simulink model "engine_model"  (R2022b)
settings: Solver=ode3  StartTime=0.0  StopTime=10  FixedStep=0.0005  RelTol=1e-3  EnableMultiTasking=on
undefined symbols (not defined in the file): sigbuilder_block
settings Model: Creator=Administrator  LastModifiedBy=Mr.Eastern
settings SolverCC: AllowMultiTaskInputOutput=on  AlgebraicLoopSolver=TrustRegion
settings DataIOCC: LimitDataPoints=on  SaveFormat=Array  SignalLoggingSaveFormat=ModelDataLogs  ReturnWorkspaceOutputs=off
settings OptimizationCC: ExpressionDepthLimit=2147483647  InitFltsAndDblsToZero=on  LifeSpan=inf
settings DebuggingCC: SaveWithParameterizedLinksMsg=none  UnderspecifiedInitializationDetection=Classic  MergeDetectMultiDrivingBlocksExec=none  SolverPrmCheckMsg=warning  FcnCallInpInsideContextMsg=warning  UnconnectedInputMsg=warning  UnconnectedOutputMsg=warning  UnconnectedLineMsg=warning  StateNameClashWarn=warning  SFUnexpectedBacktrackingDiag=warning  SFNoUnconditionalDefaultTransitionDiag=warning  SFExecutionAtInitializationDiag=none  SFMachineParentedDataDiag=warning  ArithmeticOperatorsInVariantConditions=warning
settings HardwareCC: ProdBitPerPointer=32  ProdBitPerSizeT=32  ProdBitPerPtrDiffT=32  ProdLargestAtomicFloat=None  ProdIntDivRoundTo=Undefined  ProdEndianess=Unspecified  ProdWordSize=32  ProdHWDeviceType=32-bit Generic
settings ModelReferenceCC: PropagateSignalLabelsOutOfModel=off
settings CodeAppCC: StateflowObjectComments=on
settings GRTTargetCC: TargetFcnLib=ansi_tfl_tmw.mat  TargetLangStandard=C89/C90 (ANSI)  CombineOutputUpdateFcns=off  GRTInterface=on
settings ConfigComp: CovMetricSettings=dw  CovSaveCumulativeToWorkspaceVar=on  CovSaveSingleToWorkspaceVar=on

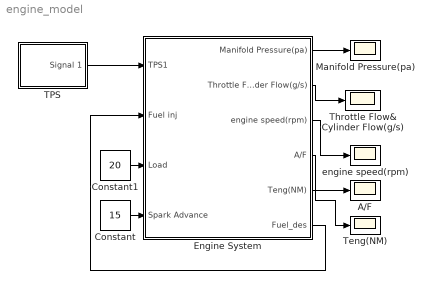
== system engine_model ==
  A/F : Scope
  Constant : Constant  Value=15
  Constant1 : Constant  Value=20
  Engine System : Subsystem
  Manifold Pressure(pa) : Scope
  TPS : Subsystem  Tag=STV Subsys  LoadFcn=sigbuilder_block('load');  StartFcn=sigbuilder_block('start');  StopFcn=sigbuilder_block('stop');  ClipboardFcn=sigbuilder_block('clipboard');  mask(Sigbuilder block){tuvar=[0:10]}
      mask help: Sigbuilder GUI
      mask init:
      | if ~strcmp(get_param(bdroot(gcb),'SimulationStatus'),'stopped') tuvar = sigbuilder_block('maskInit'); end
      settings: CopyFcn=sigbuilder_block('copy');  DeleteFcn=sigbuilder_block('delete');  ModelCloseFcn=sigbuilder_block('modelClose');  PreSaveFcn=sigbuilder_block('preSave');  PauseFcn=sigbuilder_block('pause')  ContinueFcn=sigbuilder_block('continue')  NameChangeFcn=sigbuilder_block('namechange');  OpenFcn=sigbuilder_block('open',[1520 218.5 535 348.5 ]);  CloseFcn=sigbuilder_block('close');
      mask Display: plot(0, 0, 100, 100,[2, 2, 32, 32, 2], [68, 8, 8, 68, 68],[32, 2], [38, 38], [32, 19, 2],[53, 60, 44], [32, 17, 17, 2],[16, 16, 31, 31]);txt = getActiveGroup(gcbh);text(2, 100, txt,'verticalAlignment', 'top');
  Teng(NM) : Scope
  Throttle Flow& Cylinder Flow(g/s) : Scope
  engine speed(rpm) : Scope
  wires:
  Constant/1 -> Engine System/4(Spark Advance)
  Engine System/6(Fuel_des) -> Engine System/2(Fuel inj)
  Engine System/1(Manifold Pressure(pa)) -> Manifold Pressure(pa)/1
  Engine System/2(Throttle Flow& Cylinder Flow(g/s)) -> Throttle Flow& Cylinder Flow(g/s)/1
  Engine System/3(engine speed(rpm)) -> engine speed(rpm)/1
  Engine System/4(A/F) -> A/F/1
  Engine System/5(Teng(NM)) -> Teng(NM)/1
  Constant1/1 -> Engine System/3(Load)
  TPS/1(Signal 1) -> Engine System/1(TPS1)

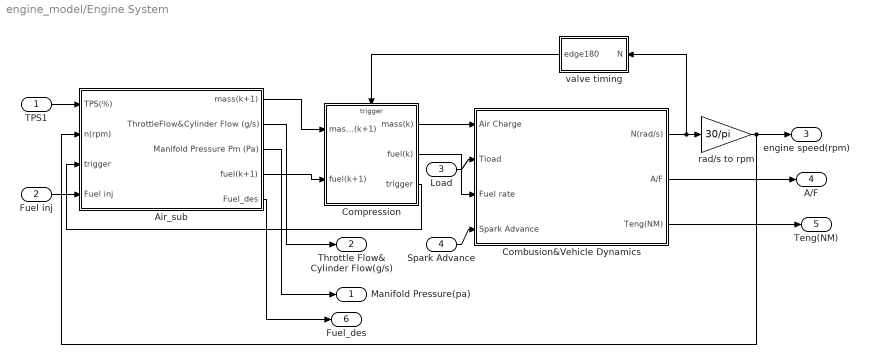
== system engine_model/Engine System ==
  TPS1 : Inport
  Fuel inj : Inport  Port=2
  Load : Inport  Port=3
  Spark Advance : Inport  Port=4
  Air_sub : Subsystem
  Combusion&Vehicle Dynamics : Subsystem
  Compression : Subsystem  TreatAsAtomicUnit=on
  rad/s to rpm : Gain  Gain=30/pi  SaturateOnIntegerOverflow=on  OutDataTypeStr=Inherit: Same as input  ParamDataTypeStr=Inherit: Same as input
  valve timing : Subsystem
  Manifold Pressure(pa) : Outport
  Throttle Flow& Cylinder Flow(g/s) : Outport  Port=2
  engine speed(rpm) : Outport  Port=3
  A/F : Outport  Port=4
  Teng(NM) : Outport  Port=5
  Fuel_des : Outport  Port=6
  wires:
  valve timing/1(edge180) -> Compression/Trigger
  Compression/1(mass(k)) -> Combusion&Vehicle Dynamics/1(Air Charge)
  Combusion&Vehicle Dynamics/1(N(rad/s)) -> valve timing/1(N), rad/s to rpm/1
  rad/s to rpm/1 -> Air_sub/2(n(rpm)), engine speed(rpm)/1
  Air_sub/1(mass(k+1)) -> Compression/1(mass(k+1))
  Load/1 -> Combusion&Vehicle Dynamics/2(Tload)
  TPS1/1 -> Air_sub/1(TPS(%))
  Combusion&Vehicle Dynamics/2(A/F) -> A/F/1
  Combusion&Vehicle Dynamics/3(Teng(NM)) -> Teng(NM)/1
  Compression/3(trigger) -> Air_sub/3(trigger)
  Air_sub/4(fuel(k+1)) -> Compression/2(fuel(k+1))
  Compression/2(fuel(k)) -> Combusion&Vehicle Dynamics/3(Fuel rate)
  Air_sub/2(ThrottleFlow&Cylinder Flow (g/s)) -> Throttle Flow& Cylinder Flow(g/s)/1
  Air_sub/3("Manifold Pressure Pm (Pa) ") -> Manifold Pressure(pa)/1
  Spark Advance/1 -> Combusion&Vehicle Dynamics/4(Spark Advance)
  Fuel inj/1 -> Air_sub/4(Fuel inj)
  Air_sub/5(Fuel_des) -> Fuel_des/1

== system engine_model/TPS ==
  Demux : Demux  Tag=STV Demux  Outputs=1
      settings: DisplayOption=none
  FromWs : FromWorkspace  Tag=STV FromWs  VariableName=tuvar  ZeroCross=off
      SigBuilderData=|
      | dataSet.timeRange = [0 10]
      | dataSet.name = 'Group 1'
      | sbobj.Groups.Name = 'Group 1'
      | sbobj.Groups.Signals.Name = 'Signal 1'
      | sbobj.Groups.Signals.XData = [0 3.54 4.02 6.64 7.58 10]
      | sbobj.Groups.Signals.YData = [20 20 81 99 42 40]
  Signal 1 : Outport  Tag=STV Outport
  wires:
  Demux/1 -> Signal 1/1
  FromWs/1 -> Demux/1

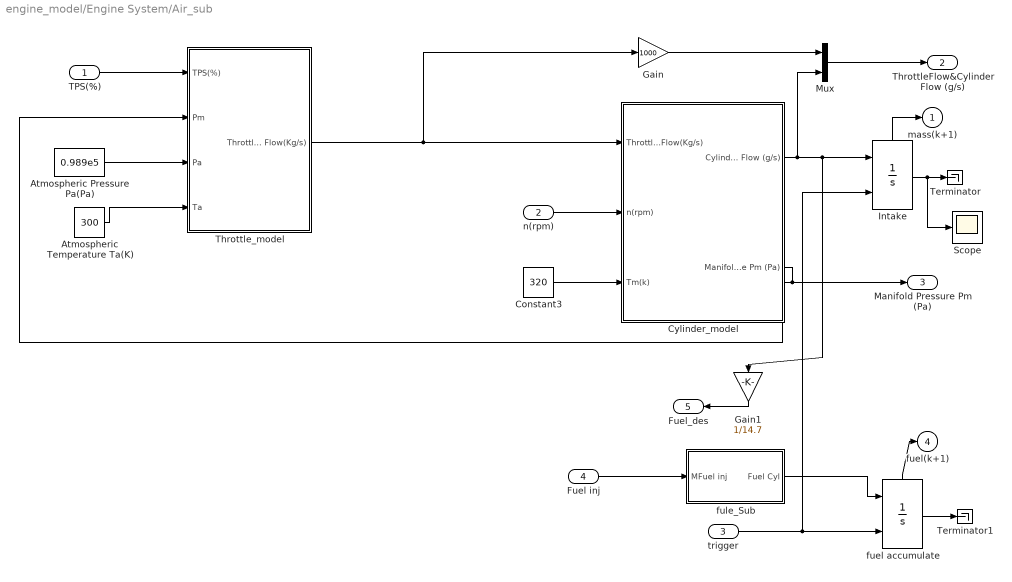
== system engine_model/Engine System/Air_sub ==
  TPS(%) : Inport
  n(rpm) : Inport  Port=2
  trigger : Inport  Port=3
  Fuel inj : Inport  Port=4
  Atmospheric Pressure Pa(Pa) : Constant  Value=0.989e5
  Atmospheric Temperature Ta(K) : Constant  Value=300
  Constant3 : Constant  Value=320
  Cylinder_model : Subsystem
  Gain : Gain  Gain=1000
  Gain1 : Gain  Gain=1/14.7
  Intake : Integrator  ExternalReset=either  ShowStatePort=on
  Mux : Mux  Inputs=2
  Scope : Scope
  Terminator : Terminator
  Terminator1 : Terminator
  Throttle_model : Subsystem
  fuel accumulate : Integrator  ExternalReset=either  ShowStatePort=on
  fule_Sub : Subsystem
  mass(k+1) : Outport  InitialOutput=0
  ThrottleFlow&Cylinder Flow (g/s) : Outport  Port=2
  "Manifold Pressure Pm (Pa) " : Outport  Port=3
  fuel(k+1) : Outport  Port=4  InitialOutput=0
  Fuel_des : Outport  Port=5
  wires:
  Cylinder_model/1(Cylinder Flow (g/s)) -> Mux/2, Intake/1, Gain1/1
  TPS(%)/1 -> Throttle_model/1(TPS(%))
  Throttle_model/1(Throttle Flow(Kg/s)) -> Cylinder_model/1(Throttle Flow(Kg/s)), Gain/1
  Atmospheric Pressure Pa(Pa)/1 -> Throttle_model/3(Pa)
  Atmospheric Temperature Ta(K)/1 -> Throttle_model/4(Ta)
  n(rpm)/1 -> Cylinder_model/2(n(rpm))
  Constant3/1 -> Cylinder_model/3(Tm(k))
  Mux/1 -> ThrottleFlow&Cylinder Flow (g/s)/1
  Cylinder_model/2(Manifold Pressure Pm (Pa)) -> Throttle_model/2(Pm), "Manifold Pressure Pm (Pa) "/1
  trigger/1 -> fuel accumulate/2, Intake/2
  Intake/1 -> Terminator/1, Scope/1
  Intake/State -> mass(k+1)/1
  fuel accumulate/1 -> Terminator1/1
  fuel accumulate/State -> fuel(k+1)/1
  Gain/1 -> Mux/1
  fule_Sub/1(Fuel Cyl) -> fuel accumulate/1
  Fuel inj/1 -> fule_Sub/1(MFuel inj)
  Gain1/1 -> Fuel_des/1

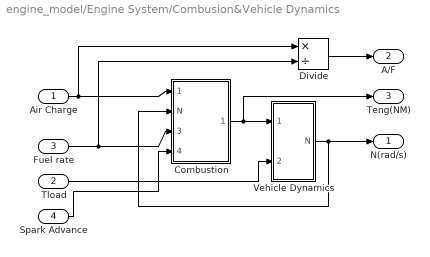
== system engine_model/Engine System/Combusion&Vehicle Dynamics ==
  Air Charge : Inport
  Tload : Inport  Port=2
  Fuel rate : Inport  Port=3
  Spark Advance : Inport  Port=4
  Combustion : Subsystem
  Divide : Product  Inputs=*/
  Vehicle Dynamics : Subsystem
  N(rad/s) : Outport
  A/F : Outport  Port=2
  Teng(NM) : Outport  Port=3
  wires:
  Vehicle Dynamics/1(N) -> Combustion/2(N), N(rad/s)/1
  Combustion/1(Torque) -> Vehicle Dynamics/1(Teng), Teng(NM)/1
  Tload/1 -> Vehicle Dynamics/2(Tload)
  Air Charge/1 -> Combustion/1(Air Charge), Divide/1
  Fuel rate/1 -> Combustion/3(Fuel rate), Divide/2
  Divide/1 -> A/F/1
  Spark Advance/1 -> Combustion/4(Spark Advance (degrees BTDC))

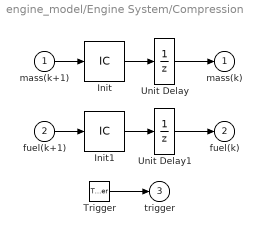
== system engine_model/Engine System/Compression ==
  mass(k+1) : Inport
  fuel(k+1) : Inport  Port=2
  Trigger : TriggerPort  TriggerType=either  VariantControl=(inherit)  ShowOutputPort=on
  Init : InitialCondition  Value=0.152
  Init1 : InitialCondition  Value=0.152
  Unit Delay : UnitDelay  InitialCondition=0.152  SampleTime=-1
  Unit Delay1 : UnitDelay  InitialCondition=0.152  SampleTime=-1
  mass(k) : Outport  InitialOutput=0.152
  fuel(k) : Outport  Port=2  InitialOutput=0.152
  trigger : Outport  Port=3  InitialOutput=-1
  wires:
  Trigger/1 -> trigger/1
  Unit Delay/1 -> mass(k)/1
  mass(k+1)/1 -> Init/1
  Unit Delay1/1 -> fuel(k)/1
  fuel(k+1)/1 -> Init1/1
  Init1/1 -> Unit Delay1/1
  Init/1 -> Unit Delay/1

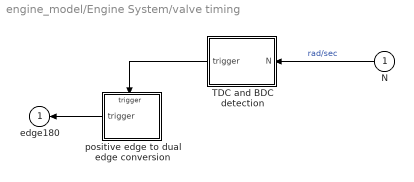
== system engine_model/Engine System/valve timing ==
  N : Inport
  TDC and BDC detection : Subsystem
  positive edge to dual edge conversion : Subsystem  TreatAsAtomicUnit=on
  edge180 : Outport  InitialOutput=-1
  wires:
  N/1 -> TDC and BDC detection/1(N)  "rad/sec"
  positive edge to dual edge conversion/1(trigger) -> edge180/1
  TDC and BDC detection/1(trigger) -> positive edge to dual edge conversion/Trigger

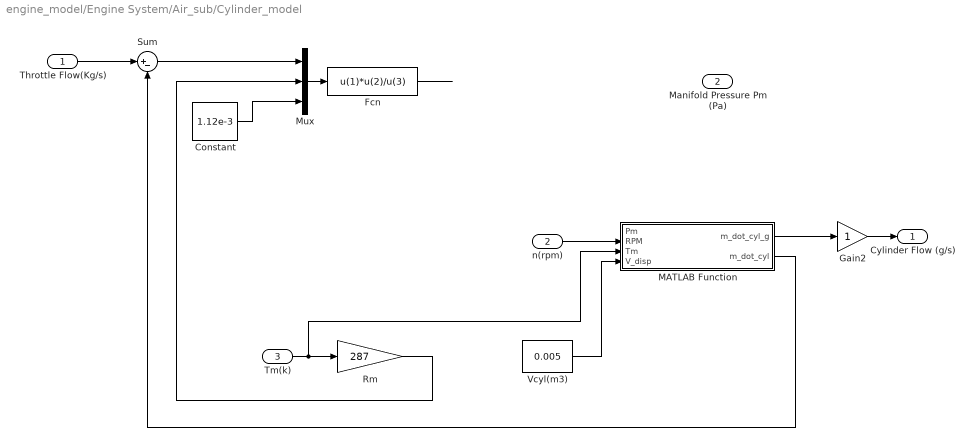
== system engine_model/Engine System/Air_sub/Cylinder_model ==
  Throttle Flow(Kg/s) : Inport
  n(rpm) : Inport  Port=2
  Tm(k) : Inport  Port=3
  Constant : Constant  Value=1.12e-3
  Fcn : Fcn  Expr=u(1)*u(2)/u(3)
  Gain2 : Gain
  MATLAB Function : MATLAB Function  TreatAsAtomicUnit=on
  Mux : Mux  Inputs=3
  Rm : Gain  Gain=287  SaturateOnIntegerOverflow=on  OutDataTypeStr=Inherit: Same as input  ParamDataTypeStr=Inherit: Same as input
  Sum : Sum  Inputs=|+-  SaturateOnIntegerOverflow=on
  Vcyl(m3) : Constant  Value=0.005
  Cylinder Flow (g/s) : Outport
  Manifold Pressure Pm (Pa) : Outport  Port=2
  wires:
  Mux/1 -> Fcn/1
  Sum/1 -> Mux/1
  Constant/1 -> Mux/3
  Throttle Flow(Kg/s)/1 -> Sum/1
  n(rpm)/1 -> MATLAB Function/2(RPM)
  Tm(k)/1 -> MATLAB Function/3(Tm), Rm/1
  Rm/1 -> Mux/2
  MATLAB Function/1(m_dot_cyl_g) -> Gain2/1
  Gain2/1 -> Cylinder Flow (g/s)/1
  Vcyl(m3)/1 -> MATLAB Function/4(V_disp)
  MATLAB Function/2(m_dot_cyl) -> Sum/2
  ? -> MATLAB Function/1(Pm), Manifold Pressure Pm (Pa)/1
  Fcn/1 -> ?

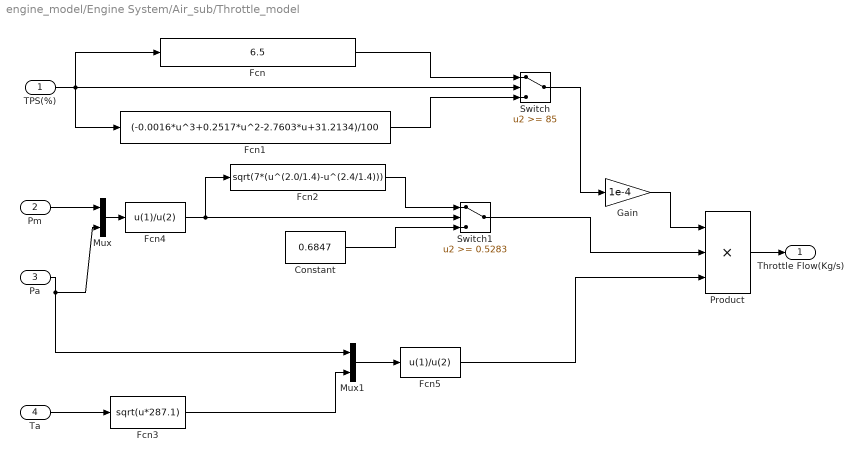
== system engine_model/Engine System/Air_sub/Throttle_model ==
  TPS(%) : Inport
  Pm : Inport  Port=2
  Pa : Inport  Port=3
  Ta : Inport  Port=4
  Constant : Constant  Value=0.6847
  Fcn : Fcn  Expr=6.5
  Fcn1 : Fcn  Expr=(-0.0016*u^3+0.2517*u^2-2.7603*u+31.2134)/100
  Fcn2 : Fcn  Expr=sqrt(7*(u^(2.0/1.4)-u^(2.4/1.4)))
  Fcn3 : Fcn  Expr=sqrt(u*287.1)
  Fcn4 : Fcn  Expr=u(1)/u(2)
  Fcn5 : Fcn  Expr=u(1)/u(2)
  Gain : Gain  Gain=1e-4  SaturateOnIntegerOverflow=on  OutDataTypeStr=Inherit: Same as input  ParamDataTypeStr=Inherit: Same as input
  Mux : Mux  Inputs=2
  Mux1 : Mux  Inputs=2
  Product : Product  Inputs=3  SaturateOnIntegerOverflow=on  OutDataTypeStr=Inherit: Same as first input
  Switch : Switch  Threshold=85  InputSameDT=off
  Switch1 : Switch  Threshold=0.5283  InputSameDT=off
  Throttle Flow(Kg/s) : Outport
  wires:
  TPS(%)/1 -> Fcn1/1, Fcn/1, Switch/2
  Fcn/1 -> Switch/1
  Fcn1/1 -> Switch/3
  Switch/1 -> Gain/1
  Gain/1 -> Product/1
  Product/1 -> Throttle Flow(Kg/s)/1
  Pm/1 -> Mux/1
  Pa/1 -> Mux1/1, Mux/2
  Fcn2/1 -> Switch1/1
  Constant/1 -> Switch1/3
  Ta/1 -> Fcn3/1
  Fcn3/1 -> Mux1/2
  Switch1/1 -> Product/2
  Mux/1 -> Fcn4/1
  Fcn4/1 -> Switch1/2, Fcn2/1
  Mux1/1 -> Fcn5/1
  Fcn5/1 -> Product/3

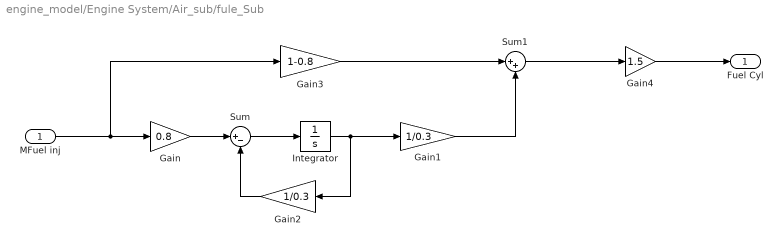
== system engine_model/Engine System/Air_sub/fule_Sub ==
  MFuel inj : Inport
  Gain : Gain  Gain=0.8  SaturateOnIntegerOverflow=on  OutDataTypeStr=Inherit: Same as input  ParamDataTypeStr=Inherit: Same as input
  Gain1 : Gain  Gain=1/0.3  SaturateOnIntegerOverflow=on  OutDataTypeStr=Inherit: Same as input  ParamDataTypeStr=Inherit: Same as input
  Gain2 : Gain  Gain=1/0.3  SaturateOnIntegerOverflow=on  OutDataTypeStr=Inherit: Same as input  ParamDataTypeStr=Inherit: Same as input
  Gain3 : Gain  Gain=1-0.8  SaturateOnIntegerOverflow=on  OutDataTypeStr=Inherit: Same as input  ParamDataTypeStr=Inherit: Same as input
  Gain4 : Gain  Gain=1.5
  Integrator : Integrator  InitialCondition=0.05
  Sum : Sum  Inputs=|+-  SaturateOnIntegerOverflow=on
  Sum1 : Sum  Inputs=|++  SaturateOnIntegerOverflow=on
  Fuel Cyl : Outport
  wires:
  MFuel inj/1 -> Gain3/1, Gain/1
  Gain/1 -> Sum/1
  Sum/1 -> Integrator/1
  Integrator/1 -> Gain2/1, Gain1/1
  Gain2/1 -> Sum/2
  Gain3/1 -> Sum1/1
  Gain1/1 -> Sum1/2
  Sum1/1 -> Gain4/1
  Gain4/1 -> Fuel Cyl/1

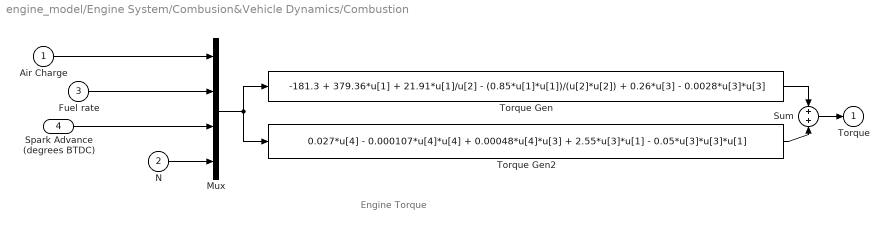
== system engine_model/Engine System/Combusion&Vehicle Dynamics/Combustion ==
  note: Engine Torque
  Air Charge : Inport
  N : Inport  Port=2
  Fuel rate : Inport  Port=3
  Spark Advance (degrees BTDC) : Inport  Port=4
  Mux : Mux
  Sum : Sum  InputSameDT=on  SaturateOnIntegerOverflow=on  OutDataTypeStr=Inherit: Same as first input
  Torque Gen : Fcn  Expr=-181.3 + 379.36*u[1] + 21.91*u[1]/u[2] - (0.85*u[1]*u[1])/(u[2]*u[2]) + 0.26*u[3] - 0.0028*u[3]*u[3]
  Torque Gen2 : Fcn  Expr=0.027*u[4] - 0.000107*u[4]*u[4] + 0.00048*u[4]*u[3] + 2.55*u[3]*u[1] - 0.05*u[3]*u[3]*u[1]
  Torque : Outport  InitialOutput=0
  wires:
  Sum/1 -> Torque/1
  Torque Gen/1 -> Sum/1
  Torque Gen2/1 -> Sum/2
  Mux/1 -> Torque Gen2/1, Torque Gen/1
  Air Charge/1 -> Mux/1
  N/1 -> Mux/4
  Spark Advance (degrees BTDC)/1 -> Mux/3
  Fuel rate/1 -> Mux/2

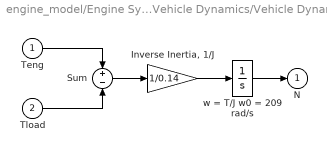
== system engine_model/Engine System/Combusion&Vehicle Dynamics/Vehicle Dynamics ==
  Teng : Inport
  Tload : Inport  Port=2
  "Inverse Inertia, 1/J" : Gain  Gain=1/0.14  SaturateOnIntegerOverflow=on  OutDataTypeStr=Inherit: Same as input  ParamDataTypeStr=Inherit: Same as input
  Sum : Sum  Inputs=+-  InputSameDT=on  SaturateOnIntegerOverflow=on  OutDataTypeStr=Inherit: Same as first input
  w = T/J w0 = 209 rad/s : Integrator  InitialCondition=150
  N : Outport  InitialOutput=0
  wires:
  Tload/1 -> Sum/2
  Teng/1 -> Sum/1
  Sum/1 -> "Inverse Inertia, 1/J"/1
  w = T/J w0 = 209 rad/s/1 -> N/1
  "Inverse Inertia, 1/J"/1 -> w = T/J w0 = 209 rad/s/1

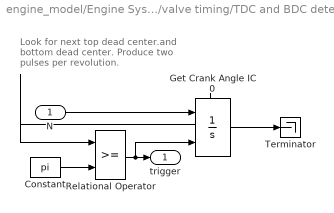
== system engine_model/Engine System/valve timing/TDC and BDC detection ==
  note: Look for next top dead center.and
      | bottom dead center.
      | Produce two pulses per revolution.
  N : Inport
  Constant : Constant  Value=pi
  Get Crank Angle IC 0 : Integrator  ExternalReset=rising  ShowStatePort=on
  Relational Operator : RelationalOperator
  Terminator : Terminator
  trigger : Outport  InitialOutput=0
  wires:
  N/1 -> Get Crank Angle IC 0/1
  Relational Operator/1 -> trigger/1, Get Crank Angle IC 0/2
  Constant/1 -> Relational Operator/2
  Get Crank Angle IC 0/State -> Relational Operator/1
  Get Crank Angle IC 0/1 -> Terminator/1

== system engine_model/Engine System/valve timing/positive edge to dual edge conversion ==
  Trigger : TriggerPort  VariantControl=(inherit)
  Gain : Gain  Gain=-1  SaturateOnIntegerOverflow=on  OutDataTypeStr=Inherit: Same as input  ParamDataTypeStr=Inherit: Same as input
  Unit Delay : UnitDelay  InitialCondition=1  SampleTime=-1
  trigger : Outport  InitialOutput=-1
  wires:
  Unit Delay/1 -> Gain/1, trigger/1
  Gain/1 -> Unit Delay/1

== matlab function engine_model/Engine System/Air_sub/Cylinder_model/MATLAB Function ==
  data: m_dot_cyl_g output; Pm input; m_dot_cyl output; RPM input; Tm input; V_disp input
function [m_dot_cyl_g,m_dot_cyl] = fcn(Pm, RPM, Tm, V_disp)
    % 输入:
    % Pm: 歧管压力 (Pa)
    % RPM: 转速
    % Tm: 进气温度 (K)
    % V_disp: 单缸排量 (m3) - 来自原来的 Vcyl 模块

    % --- 转子发动机特性参数 ---
    R = 287; % 气体常数
    % 转子充气效率模型 (随转速变化)
    eta_vol = 0.85 + 0.1 * sin(RPM/8000 * pi); 
    
    % --- 计算进入气缸的空气流量 (kg/s) ---
    % 理想气体密度 rho = P / (RT)
    rho = Pm / (R * Tm);
    
    % 流量公式: m_dot = eta * V_disp * rho * (RPM/60) * (点火频次系数)
    % 对于双转子，相当于排量每转一次完全吸气一次 (系数取1或0.5视具体定义，这里取1保证流量够大)
    m_dot_cyl = eta_vol * V_disp * rho * (RPM/60);
    
    % --- 转换为 g/s (因为Gain2后面需要g/s) ---
    m_dot_cyl_g = m_dot_cyl * 1000;
end
